simulink model "QpskFFRC"  (R2015a)
settings: Solver=ode45  StartTime=0.0  StopTime=Inf  RelTol=1e-3
libraries: commnoisgen2 x2, commdigbbndpm3 x2, commsink2 x1, commchan3 x1, commrandsrc2 x1
settings Model: Creator=konstantis  LastModifiedBy=konstantis

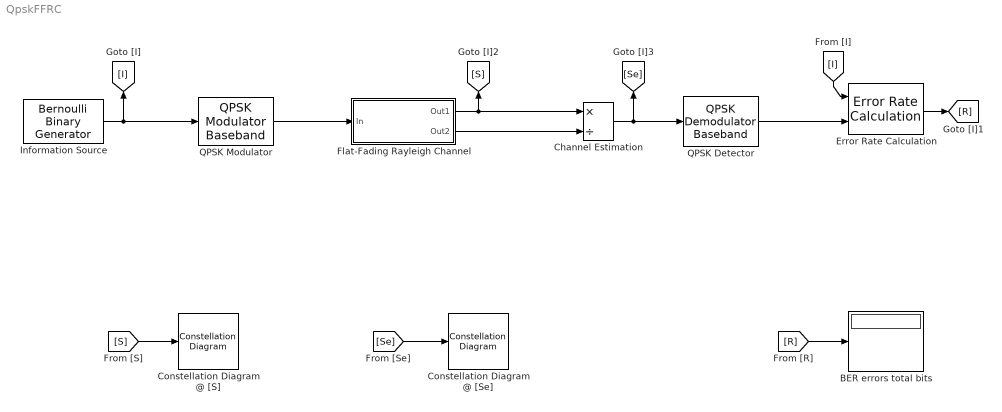
== system QpskFFRC ==
  BER errors total bits : Display
      settings: Format=short_e
  Channel Estimation : Product  Inputs=*/
  Constellation Diagram @ [S] : ConstellationDiagram
  Constellation Diagram @ [Se] : ConstellationDiagram
  Error Rate Calculation : commsink2/Error Rate Calculation  N=0  st_delay=0  cp_mode=Entire frame  subframe=[]  PMode=Port  WsName=ErrorVec  RsMode2=off  stop=off  numErr=100  maxBits=1e6
  Flat-Fading Rayleigh Channel : Subsystem
  Information Source : commrandsrc2/Bernoulli Binary Generator  P=0.5  seed=61  Ts=.001  frameBased=on  sampPerFrame=1000  orient=off  outDataType=double
  QPSK Detector : commdigbbndpm3/QPSK Demodulator Baseband  Ph=pi/4  Dec=Gray  OutType=Bit  DecType=Hard decision  VarSource=Dialog  Variance=1  outDtype1=Inherit via internal rule  outDtype2=Inherit via internal rule  derotateFactorWordLen=16
  QPSK Modulator : commdigbbndpm3/QPSK Modulator Baseband  InType=Bit  Enc=Gray  Ph=pi/4  outDtype=double  outWordLen=16  outUDDataType=sfix(16)  outFracLenMode=Best precision  outFracLen=15
  wires:
  Information Source/1 -> [I], QPSK Modulator/1
  QPSK Detector/1 -> Error Rate Calculation/2
  QPSK Modulator/1 -> Flat-Fading Rayleigh Channel/1(In)
  Flat-Fading Rayleigh Channel/1(Out1) -> Channel Estimation/1, [S]
  Flat-Fading Rayleigh Channel/2(Out2) -> Channel Estimation/2
  Channel Estimation/1 -> [Se], QPSK Detector/1
  [I] -> Error Rate Calculation/1
  Error Rate Calculation/1 -> [R]
  [R] -> BER errors total bits/1
  [S] -> Constellation Diagram @ [S]/1
  [Se] -> Constellation Diagram @ [Se]/1

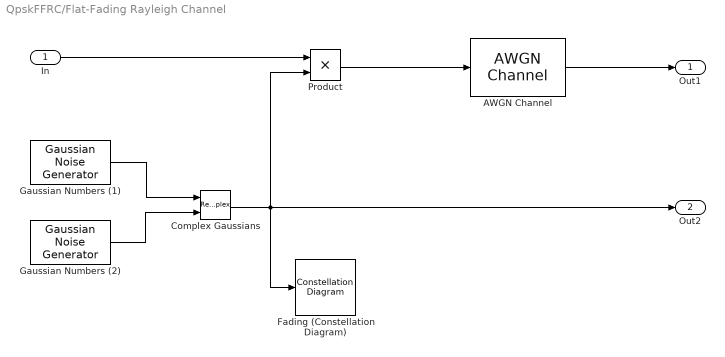
== system QpskFFRC/Flat-Fading Rayleigh Channel ==
  In : Inport
  AWGN Channel : commchan3/AWGN Channel  InputProcessing=Columns as channels (frame based)  seed=67  noiseMode="Signal to noise ratio  (SNR)"  EbNodB=10  EsNodB=10  SNRdB=23  bitsPerSym=2  Ps=1  Tsym=1  variance=1
  Complex Gaussians : RealImagToComplex
  Fading (Constellation Diagram) : ConstellationDiagram
  Gaussian Numbers (1) : commnoisgen2/Gaussian Noise Generator  m=0  d=1/2  s=41  Ts=.001  frameBased=on  sampPerFrame=500  orient=off  outDataType=double
  Gaussian Numbers (2) : commnoisgen2/Gaussian Noise Generator  m=0  d=1/2  s=2^31  Ts=.001  frameBased=on  sampPerFrame=500  orient=off  outDataType=double
  Product : Product
  Out1 : Outport
  Out2 : Outport  Port=2
  wires:
  Gaussian Numbers (1)/1 -> Complex Gaussians/1
  Gaussian Numbers (2)/1 -> Complex Gaussians/2
  In/1 -> Product/1
  Complex Gaussians/1 -> Fading (Constellation Diagram)/1, Out2/1, Product/2
  Product/1 -> AWGN Channel/1
  AWGN Channel/1 -> Out1/1
